simulink subsystem "controller"  (R2025b)
settings: Solver=VariableStepAuto  StartTime=0.0  StopTime=10.0  RelTol=1e-3
undefined symbols (not defined in the file or in its folder): dt_control, dt_data
libraries: simulink x1
settings Model: Creator=koryh  LastModifiedBy=kjhaydon

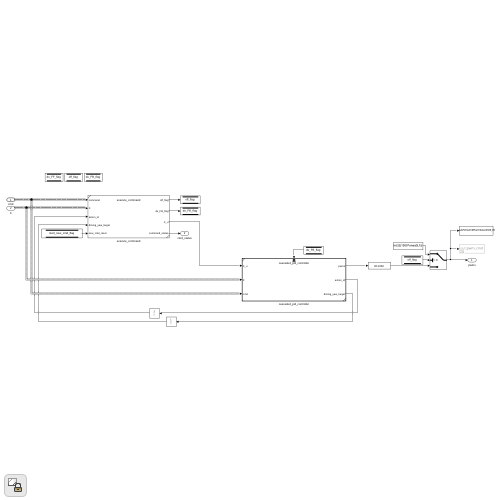
[thumbnail: Simulink's stored preview of the top-level diagram]
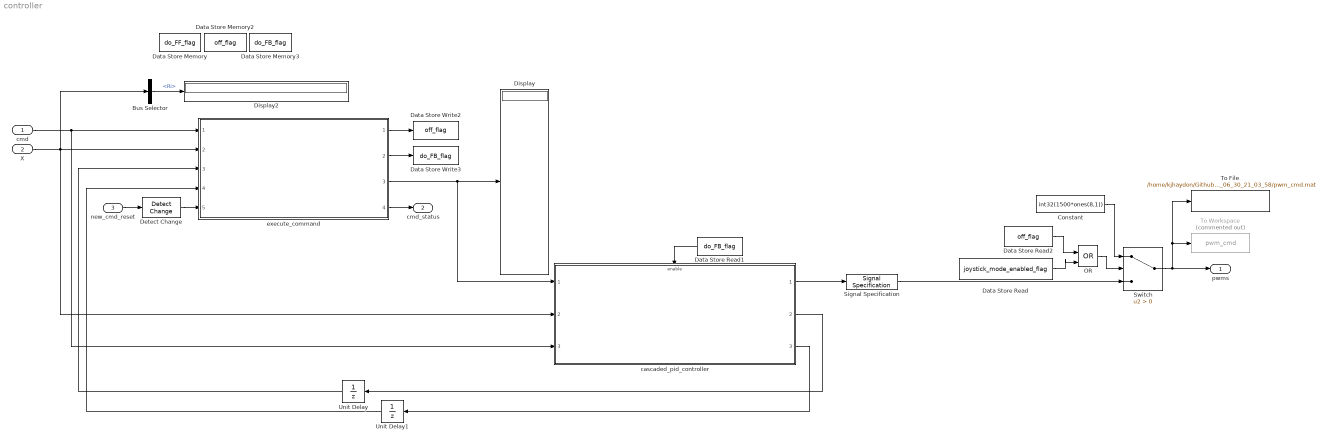
== system controller ==
  cmd : Inport  OutDataTypeStr=Bus: cmd_bus  SampleTime=dt_control
      settings: VarSizeSig=Yes
  X : Inport  Port=2  SampleTime=dt_control
  new_cmd_reset : Inport  Port=3
  Bus Selector : BusSelector  OutputSignals=Ri
  Constant : Constant  Value=int32(1500*ones(8,1))
  Data Store Memory : DataStoreMemory  DataStoreName=do_FF_flag  WriteAfterWriteMsg=warning  ShowAdditionalParam=off
  Data Store Memory2 : DataStoreMemory  DataStoreName=off_flag  WriteAfterWriteMsg=warning  ShowAdditionalParam=off
  Data Store Memory3 : DataStoreMemory  DataStoreName=do_FB_flag  WriteAfterWriteMsg=warning  ShowAdditionalParam=off
  Data Store Read : DataStoreRead  DataStoreName=joystick_mode_enabled_flag  IndexOptions=Index vector (dialog)  Indices=1  OutputSizes=1
  Data Store Read1 : DataStoreRead  DataStoreName=do_FB_flag  IndexOptions=Index vector (dialog)  Indices=1  OutputSizes=1
  Data Store Read2 : DataStoreRead  DataStoreName=off_flag  IndexOptions=Index vector (dialog)  Indices=1  OutputSizes=1
  Data Store Write2 : DataStoreWrite  DataStoreName=off_flag  IndexOptions=Index vector (dialog)  Indices=1  OutputSizes=1
  Data Store Write3 : DataStoreWrite  DataStoreName=do_FB_flag  IndexOptions=Index vector (dialog)  Indices=1  OutputSizes=1
  Detect Change : simulink/Logic and Bit Operations/Detect Change  vinit=0  OutDataTypeStr=boolean
  Display : Display
  Display2 : Display
  OR : Logic  Operator=OR  IconShape=distinctive  AllPortsSameDT=off  OutDataTypeStr=boolean
  Signal Specification : SignalSpecification  OutDataTypeStr=int32
  Switch : Switch  Criteria=u2 > Threshold  SaturateOnIntegerOverflow=off  InputSameDT=off
  To File : ToFile  Filename=/home/kjhaydon/Github/Robosub/SimulinkPlant/data/2026_06_30_21_03_58/pwm_cmd.mat  MatrixName=pwm_cmd  SaveFormat=Timeseries  SampleTime=dt_data
  To Workspace : ToWorkspace  Commented=on  VariableName=pwm_cmd  SaveFormat=Timeseries  SampleTime=dt_data
  Unit Delay : UnitDelay  SampleTime=dt_control  HasFrameUpgradeWarning=on
  Unit Delay1 : UnitDelay  SampleTime=dt_control  HasFrameUpgradeWarning=on
  cascaded_pid_controller : Subsystem  ReferencedSubsystem=cascaded_pid_controller
  execute_command : Subsystem  ReferencedSubsystem=execute_command
  pwms : Outport
  cmd_status : Outport  Port=2  SampleTime=dt_control
  wires:
  X/1 -> cascaded_pid_controller/2, execute_command/2, Bus Selector/1
  Switch/1 -> pwms/1, To File/1, To Workspace/1
  Data Store Read1/1 -> cascaded_pid_controller/Enable
  Constant/1 -> Switch/1
  cascaded_pid_controller/1 -> Signal Specification/1
  Signal Specification/1 -> Switch/3
  cascaded_pid_controller/2 -> Unit Delay/1
  Unit Delay/1 -> execute_command/3
  cascaded_pid_controller/3 -> Unit Delay1/1
  execute_command/3 -> cascaded_pid_controller/1, Display/1
  execute_command/1 -> Data Store Write2/1
  execute_command/2 -> Data Store Write3/1
  execute_command/4 -> cmd_status/1
  cmd/1 -> execute_command/1, cascaded_pid_controller/3
  Unit Delay1/1 -> execute_command/4
  OR/1 -> Switch/2
  Data Store Read/1 -> OR/2
  Data Store Read2/1 -> OR/1
  new_cmd_reset/1 -> Detect Change/1
  Bus Selector/1 -> Display2/1  "<Ri>"
  Detect Change/1 -> execute_command/5
